simulink model "code_gen_HeadingHold"  (Simulink 7.5)
settings: Solver=FixedStepDiscrete  SolverMode=SingleTasking  StartTime=0.0  StopTime=10.0  FixedStep=0.01  RelTol=1e-3
InitFcn:
  | boat_constants
values from neighbouring files (symbols this model uses):
  figure8_waypoints = int32([ ... (first row only)    [boat_constants.m]
  OC2max = 49999    [boat_constants.m]    (also in simulation_constants.m)
  sampling_waypoints = int32([ ... (first row only)    [boat_constants.m]
  T_step = 0.01    [boat_constants.m]    (also in common.m)
  test_waypoints = int32([ ... (first row only)    [boat_constants.m]
undefined symbols (not defined in the file or in its folder): clearGpsData, clearSensorData, cpInitCommunications, DataEEInitAndClear, DataEEWrite, DiscIntNeverNeededParam, ecan1_buffered_transmit_matlab, ecan1_error_status_matlab, ecan1_init, ecan1_receive_matlab, getGpsData, getSensorData, Init_onlyOnce, Init_Reset, initCalibrationRange, initGps, processNewCommData, processNewGpsData, setHilMode, u1, u2, uart1EnqueueStateData, uart2EnqueueActuatorData, y1
libraries: simulink x85, dsPICdrivers x44, uSimLib x6, simulink_need_slupdate x4, aerolibconvert2 x2
(part 5 of 6)

== system code_gen_HeadingHold/Controller/Autonomous Controller/Throttle Command/Mux Everything/Build speed command ==
  CC : Inport  OutDataType=sfix(16)  OutScaling=2^0
  Constant : Constant  OutDataTypeMode=uint8  OutDataType=sfix(16)  OutScaling=2^0  OutDataTypeStr=uint8
  Constant1 : Constant  Value=0  OutDataTypeMode=uint8  OutDataType=sfix(16)  OutScaling=2^0  OutDataTypeStr=uint8
  Constant2 : Constant  Value=0  OutDataTypeMode=uint8  OutDataType=sfix(16)  OutScaling=2^0  OutDataTypeStr=uint8
  Constant3 : Constant  Value=5  OutDataTypeMode=uint8  OutDataType=sfix(16)  OutScaling=2^0  OutDataTypeStr=uint8
  Mux : Mux  Inputs=5
  uint16 to uchar : Subsystem  AncestorBlock=uSimLib/Conversions/uint16 to uchar
  msg : Outport  OutDataType=sfix(16)  OutScaling=2^0
  wires:
  uint16 to uchar/1(uchar) -> Mux/3
  Constant/1 -> Mux/1
  Constant3/1 -> Mux/2
  Mux/1 -> msg/1
  Constant1/1 -> Mux/4
  Constant2/1 -> Mux/5
  CC/1 -> uint16 to uchar/1(ushort)

== system code_gen_HeadingHold/Controller/RC Inputs/Map PWM values to Actuator Signals/Throttle Command/Mux Everything ==
  speed : Inport  OutDataType=sfix(16)  OutScaling=2^0
  enable : Inport  Port=2  OutDataType=sfix(16)  OutScaling=2^0
  Throttle : Inport  Port=3  OutDataType=sfix(16)  OutScaling=2^0
  0x300 : Constant  Value=768  OutDataTypeMode=uint32  OutDataType=sfix(16)  OutScaling=2^0  OutDataTypeStr=uint32
  0x301 : Constant  Value=769  OutDataTypeMode=uint32  OutDataType=sfix(16)  OutScaling=2^0  OutDataTypeStr=uint32
  Build speed command : Subsystem
  Enable motor : Constant  Value=[0 0 0 0 32 0]  OutDataTypeMode=uint8  OutDataType=sfix(16)  OutScaling=2^0  OutDataTypeStr=uint8
  Message Length1 : Probe  ProbeSampleTime=off  ProbeComplexSignal=off  ProbeWidthDataType=uint8
  Switch : Switch  Criteria=u2 ~= 0  Threshold=1
  Switch1 : Switch  Criteria=u2 ~= 0  OutDataType=fixdt(1, 16)  OutScaling=2^0
  iden : Outport  OutDataType=sfix(16)  OutScaling=2^0
  data : Outport  Port=2  OutDataType=sfix(16)  OutScaling=2^0
  size : Outport  Port=3  OutDataType=sfix(16)  OutScaling=2^0
  trig : Outport  Port=4  OutDataType=sfix(16)  OutScaling=2^0
  wires:
  Throttle/1 -> Build speed command/1(CC)
  Message Length1/1 -> size/1
  0x301/1 -> Switch/3
  Switch1/1 -> Message Length1/1, data/1
  0x300/1 -> Switch/1
  enable/1 -> Switch/2, Switch1/2
  speed/1 -> trig/1
  Enable motor/1 -> Switch1/1
  Build speed command/1(msg) -> Switch1/3
  Switch/1 -> iden/1

== system code_gen_HeadingHold/Controller/RC Inputs/Map PWM values to Actuator Signals/Throttle Command/Trigger Events ==
  Throttle : Inport  OutDataType=sfix(16)  OutScaling=2^0
  Data Type Conversion3 : DataTypeConversion  OutDataTypeMode=boolean  OutDataType=sfix(16)  OutScaling=2^0  OutDataTypeStr=boolean
  Detect Change : simulink/Logic and Bit Operations/Detect Change  SystemSampleTime=-1  vinit=0
  Shift Arithmetic : simulink/Logic and Bit Operations/Shift Arithmetic  SystemSampleTime=-1  nBitShiftRight=2  nBinPtShiftRight=0
  Weighted Moving Average : simulink_need_slupdate/Weighted Moving Average  mgainval=[.5 .5]  vinit=0.0  samptime=-1  OutDataTypeStr=Inherit: Inherit via back propagation  OutDataType=sfix(16)  OutScaling=2^-10  DoSatur=off  GainDataType=uint(16)  MatRadixGroup=Best Precision: Matrix-wise  GainScaling=2^-10
  Change Speed : Outport  OutDataType=sfix(16)  OutScaling=2^0
  wires:
  Throttle/1 -> Shift Arithmetic/1
  Detect Change/1 -> Data Type Conversion3/1
  Data Type Conversion3/1 -> Change Speed/1
  Weighted Moving Average/1 -> Detect Change/1
  Shift Arithmetic/1 -> Weighted Moving Average/1

== system code_gen_HeadingHold/Controller/Radio Control Inputs1/Calibration/Update range from input/If Action Subsystem ==
  In1 : Inport  OutDataType=fixdt(1, 16)  OutScaling=2^0
  Action Port : ActionPort  ActionType=then
  Out1 : Outport  OutDataType=fixdt(1, 16)  OutScaling=2^0
  wires:
  In1/1 -> Out1/1

== system code_gen_HeadingHold/Controller/Radio Control Inputs1/Calibration/Update range from input/If Action Subsystem1 ==
  In1 : Inport  OutDataType=fixdt(1, 16)  OutScaling=2^0
  Action Port : ActionPort  ActionType=else
  Out1 : Outport  OutDataType=fixdt(1, 16)  OutScaling=2^0
  wires:
  In1/1 -> Out1/1

== system code_gen_HeadingHold/Controller/Radio Control Inputs1/Calibration/Update range from input/If Action Subsystem2 ==
  In1 : Inport  OutDataType=fixdt(1, 16)  OutScaling=2^0
  Action Port : ActionPort  ActionType=then
  Out1 : Outport  OutDataType=fixdt(1, 16)  OutScaling=2^0
  wires:
  In1/1 -> Out1/1

== system code_gen_HeadingHold/Controller/Radio Control Inputs1/Calibration/Update range from input/If Action Subsystem3 ==
  In1 : Inport  OutDataType=fixdt(1, 16)  OutScaling=2^0
  Action Port : ActionPort  ActionType=else
  Out1 : Outport  OutDataType=fixdt(1, 16)  OutScaling=2^0
  wires:
  In1/1 -> Out1/1

== system code_gen_HeadingHold/Controller/Radio Control Inputs1/Calibration/Update range from input1/If Action Subsystem ==
  In1 : Inport  OutDataType=fixdt(1, 16)  OutScaling=2^0
  Action Port : ActionPort  ActionType=then
  Out1 : Outport  OutDataType=fixdt(1, 16)  OutScaling=2^0
  wires:
  In1/1 -> Out1/1

== system code_gen_HeadingHold/Controller/Radio Control Inputs1/Calibration/Update range from input1/If Action Subsystem1 ==
  In1 : Inport  OutDataType=fixdt(1, 16)  OutScaling=2^0
  Action Port : ActionPort  ActionType=else
  Out1 : Outport  OutDataType=fixdt(1, 16)  OutScaling=2^0
  wires:
  In1/1 -> Out1/1

== system code_gen_HeadingHold/Controller/Radio Control Inputs1/Calibration/Update range from input1/If Action Subsystem2 ==
  In1 : Inport  OutDataType=fixdt(1, 16)  OutScaling=2^0
  Action Port : ActionPort  ActionType=then
  Out1 : Outport  OutDataType=fixdt(1, 16)  OutScaling=2^0
  wires:
  In1/1 -> Out1/1

== system code_gen_HeadingHold/Controller/Radio Control Inputs1/Calibration/Update range from input1/If Action Subsystem3 ==
  In1 : Inport  OutDataType=fixdt(1, 16)  OutScaling=2^0
  Action Port : ActionPort  ActionType=else
  Out1 : Outport  OutDataType=fixdt(1, 16)  OutScaling=2^0
  wires:
  In1/1 -> Out1/1

== system code_gen_HeadingHold/Controller/Radio Control Inputs1/Calibration/Update range from input2/If Action Subsystem ==
  In1 : Inport  OutDataType=fixdt(1, 16)  OutScaling=2^0
  Action Port : ActionPort  ActionType=then
  Out1 : Outport  OutDataType=fixdt(1, 16)  OutScaling=2^0
  wires:
  In1/1 -> Out1/1

== system code_gen_HeadingHold/Controller/Radio Control Inputs1/Calibration/Update range from input2/If Action Subsystem1 ==
  In1 : Inport  OutDataType=fixdt(1, 16)  OutScaling=2^0
  Action Port : ActionPort  ActionType=else
  Out1 : Outport  OutDataType=fixdt(1, 16)  OutScaling=2^0
  wires:
  In1/1 -> Out1/1

== system code_gen_HeadingHold/Controller/Radio Control Inputs1/Calibration/Update range from input2/If Action Subsystem2 ==
  In1 : Inport  OutDataType=fixdt(1, 16)  OutScaling=2^0
  Action Port : ActionPort  ActionType=then
  Out1 : Outport  OutDataType=fixdt(1, 16)  OutScaling=2^0
  wires:
  In1/1 -> Out1/1

== system code_gen_HeadingHold/Controller/Radio Control Inputs1/Calibration/Update range from input2/If Action Subsystem3 ==
  In1 : Inport  OutDataType=fixdt(1, 16)  OutScaling=2^0
  Action Port : ActionPort  ActionType=else
  Out1 : Outport  OutDataType=fixdt(1, 16)  OutScaling=2^0
  wires:
  In1/1 -> Out1/1

== system code_gen_HeadingHold/Controller/Radio Control Inputs1/Detect calibration trigger/State outputs/If Action Subsystem1 ==
  Action Port : ActionPort  ActionType=then
  Constant1 : Constant  Value=false  OutDataType=fixdt(1, 16)  OutScaling=2^0  OutDataTypeStr=Inherit: Inherit via back propagation
  LED : Outport  OutDataType=fixdt(1, 16)  OutScaling=2^0  InitialOutput=false
  wires:
  Constant1/1 -> LED/1

== system code_gen_HeadingHold/Controller/Radio Control Inputs1/Detect calibration trigger/State outputs/If Action Subsystem2 ==
  Action Port : ActionPort  ActionType=else
  Constant1 : Constant  Value=false  OutDataType=fixdt(1, 16)  OutScaling=2^0  OutDataTypeStr=Inherit: Inherit via back propagation
  LED : Outport  OutDataType=fixdt(1, 16)  OutScaling=2^0  InitialOutput=false
  wires:
  Constant1/1 -> LED/1

== system code_gen_HeadingHold/Controller/Radio Control Inputs1/Detect calibration trigger/State outputs/If Action Subsystem3 ==
  Pulse : Inport
  Action Port : ActionPort  ActionType=elseif
  LED : Outport  OutDataType=fixdt(1, 16)  OutScaling=2^0  InitialOutput=false
  wires:
  Pulse/1 -> LED/1

== system code_gen_HeadingHold/Controller/Radio Control Inputs1/Detect calibration trigger/State outputs/If Action Subsystem4 ==
  Action Port : ActionPort  ActionType=elseif
  Constant1 : Constant  Value=true  OutDataType=fixdt(1, 16)  OutScaling=2^0  OutDataTypeStr=Inherit: Inherit via back propagation
  LED : Outport  OutDataType=fixdt(1, 16)  OutScaling=2^0  InitialOutput=false
  wires:
  Constant1/1 -> LED/1

== system code_gen_HeadingHold/Controller/Radio Control Inputs1/If Action Subsystem1/Add 8% center deadband/If Action Subsystem ==
  In1 : Inport  OutDataType=fixdt(1, 16)  OutScaling=2^0
  Action Port : ActionPort  ActionType=else
  Out1 : Outport  OutDataType=fixdt(1, 16)  OutScaling=2^0
  wires:
  In1/1 -> Out1/1

== system code_gen_HeadingHold/Controller/Radio Control Inputs1/If Action Subsystem1/Add 8% center deadband/If Action Subsystem1 ==
  Action Port : ActionPort  ActionType=then
  Constant : Constant  Value=0  OutDataType=fixdt(1, 16)  OutScaling=2^0  OutDataTypeStr=Inherit: Inherit via back propagation
  Out1 : Outport  OutDataType=fixdt(1, 16)  OutScaling=2^0  InitialOutput=50
  wires:
  Constant/1 -> Out1/1

== system code_gen_HeadingHold/Controller/Radio Control Inputs1/If Action Subsystem3/Add 5% deadband about 0/If Action Subsystem ==
  In1 : Inport  OutDataType=fixdt(1, 16)  OutScaling=2^0
  Action Port : ActionPort  ActionType=else
  Out1 : Outport  OutDataType=fixdt(1, 16)  OutScaling=2^0
  wires:
  In1/1 -> Out1/1

== system code_gen_HeadingHold/Controller/Radio Control Inputs1/If Action Subsystem3/Add 5% deadband about 0/If Action Subsystem1 ==
  Action Port : ActionPort  ActionType=then
  Constant : Constant  Value=0  OutDataType=fixdt(1, 16)  OutScaling=2^0  OutDataTypeStr=Inherit: Inherit via back propagation
  Out1 : Outport  OutDataType=fixdt(1, 16)  OutScaling=2^0  InitialOutput=0
  wires:
  Constant/1 -> Out1/1

== system code_gen_HeadingHold/Controller/Radio Control Inputs1/If Action Subsystem5/Add 8% center deadband/If Action Subsystem ==
  In1 : Inport  OutDataType=fixdt(1, 16)  OutScaling=2^0
  Action Port : ActionPort  ActionType=else
  Out1 : Outport  OutDataType=fixdt(1, 16)  OutScaling=2^0
  wires:
  In1/1 -> Out1/1

== system code_gen_HeadingHold/Controller/Radio Control Inputs1/If Action Subsystem5/Add 8% center deadband/If Action Subsystem1 ==
  Action Port : ActionPort  ActionType=then
  Constant : Constant  Value=500  OutDataType=fixdt(1, 16)  OutScaling=2^0  OutDataTypeStr=Inherit: Inherit via back propagation
  Out1 : Outport  OutDataType=fixdt(1, 16)  OutScaling=2^0  InitialOutput=50
  wires:
  Constant/1 -> Out1/1

== system code_gen_HeadingHold/Controller/Split trackCommand to singular commands/Countdown timer for trigger/State transitions/Null transition (necessary for merge block) ==
  Action Port : ActionPort  ActionType=else
  Constant1 : Constant  Value=false  OutDataTypeMode=boolean  OutDataType=fixdt(1, 16)  OutScaling=2^0  OutDataTypeStr=boolean
  Constant3 : Constant  Value=false  OutDataTypeMode=boolean  OutDataType=fixdt(1, 16)  OutScaling=2^0  OutDataTypeStr=boolean
  startTimer : Outport  OutDataType=fixdt(1, 16)  OutScaling=2^0  InitialOutput=false
  trigger : Outport  Port=2  OutDataType=fixdt(1, 16)  OutScaling=2^0  InitialOutput=false
  wires:
  Constant3/1 -> startTimer/1
  Constant1/1 -> trigger/1

== system code_gen_HeadingHold/Controller/Split trackCommand to singular commands/Countdown timer for trigger/State transitions/Transition from 0 to 1 ==
  Action Port : ActionPort  ActionType=then
  Constant : Constant  OutDataType=fixdt(1, 16)  OutScaling=2^0  OutDataTypeStr=Inherit: Inherit via back propagation
  Constant2 : Constant  Value=true  OutDataTypeMode=boolean  OutDataType=fixdt(1, 16)  OutScaling=2^0  OutDataTypeStr=boolean
  Constant3 : Constant  Value=false  OutDataTypeMode=boolean  OutDataType=fixdt(1, 16)  OutScaling=2^0  OutDataTypeStr=boolean
  Data Store Write : DataStoreWrite  DataStoreName=timerState  SampleTime=-1
  startTimer : Outport  OutDataType=fixdt(1, 16)  OutScaling=2^0  InitialOutput=true
  trigger : Outport  Port=2  OutDataType=fixdt(1, 16)  OutScaling=2^0  InitialOutput=true
  wires:
  Constant/1 -> Data Store Write/1
  Constant2/1 -> startTimer/1
  Constant3/1 -> trigger/1

== system code_gen_HeadingHold/Controller/Split trackCommand to singular commands/Countdown timer for trigger/State transitions/Transition from 1 to 0 ==
  Action Port : ActionPort  ActionType=elseif
  Constant : Constant  Value=0  OutDataType=fixdt(1, 16)  OutScaling=2^0  OutDataTypeStr=Inherit: Inherit via back propagation
  Constant1 : Constant  Value=false  OutDataTypeMode=boolean  OutDataType=fixdt(1, 16)  OutScaling=2^0  OutDataTypeStr=boolean
  Constant3 : Constant  Value=false  OutDataTypeMode=boolean  OutDataType=fixdt(1, 16)  OutScaling=2^0  OutDataTypeStr=boolean
  Data Store Write : DataStoreWrite  DataStoreName=timerState  SampleTime=-1
  startTimer : Outport  OutDataType=fixdt(1, 16)  OutScaling=2^0  InitialOutput=false
  trigger : Outport  Port=2  OutDataType=fixdt(1, 16)  OutScaling=2^0  InitialOutput=false
  wires:
  Constant/1 -> Data Store Write/1
  Constant3/1 -> startTimer/1
  Constant1/1 -> trigger/1

== system code_gen_HeadingHold/Controller/Split trackCommand to singular commands/Countdown timer for trigger/State transitions/Transition from 1 to 2 ==
  Action Port : ActionPort  ActionType=elseif
  Constant : Constant  Value=2  OutDataType=fixdt(1, 16)  OutScaling=2^0  OutDataTypeStr=Inherit: Inherit via back propagation
  Constant1 : Constant  Value=true  OutDataTypeMode=boolean  OutDataType=fixdt(1, 16)  OutScaling=2^0  OutDataTypeStr=boolean
  Constant3 : Constant  Value=false  OutDataTypeMode=boolean  OutDataType=fixdt(1, 16)  OutScaling=2^0  OutDataTypeStr=boolean
  Data Store Write : DataStoreWrite  DataStoreName=timerState  SampleTime=-1
  startTimer : Outport  OutDataType=fixdt(1, 16)  OutScaling=2^0  InitialOutput=false
  trigger : Outport  Port=2  OutDataType=fixdt(1, 16)  OutScaling=2^0  InitialOutput=false
  wires:
  Constant/1 -> Data Store Write/1
  Constant3/1 -> startTimer/1
  Constant1/1 -> trigger/1

== system code_gen_HeadingHold/Controller/Split trackCommand to singular commands/Countdown timer for trigger/State transitions/Transition from 2 to 0 ==
  Action Port : ActionPort  ActionType=elseif
  Constant : Constant  Value=0  OutDataType=fixdt(1, 16)  OutScaling=2^0  OutDataTypeStr=Inherit: Inherit via back propagation
  Constant1 : Constant  Value=false  OutDataTypeMode=boolean  OutDataType=fixdt(1, 16)  OutScaling=2^0  OutDataTypeStr=boolean
  Constant3 : Constant  Value=false  OutDataTypeMode=boolean  OutDataType=fixdt(1, 16)  OutScaling=2^0  OutDataTypeStr=boolean
  Data Store Write : DataStoreWrite  DataStoreName=timerState  SampleTime=-1
  startTimer : Outport  OutDataType=fixdt(1, 16)  OutScaling=2^0  InitialOutput=false
  trigger : Outport  Port=2  OutDataType=fixdt(1, 16)  OutScaling=2^0  InitialOutput=false
  wires:
  Constant/1 -> Data Store Write/1
  Constant3/1 -> startTimer/1
  Constant1/1 -> trigger/1

== system code_gen_HeadingHold/Controller/Split trackCommand to singular commands/Countdown timer for trigger1/State transitions/Null transition (necessary for merge block) ==
  Action Port : ActionPort  ActionType=else
  Constant1 : Constant  Value=false  OutDataTypeMode=boolean  OutDataType=fixdt(1, 16)  OutScaling=2^0  OutDataTypeStr=boolean
  Constant3 : Constant  Value=false  OutDataTypeMode=boolean  OutDataType=fixdt(1, 16)  OutScaling=2^0  OutDataTypeStr=boolean
  startTimer : Outport  OutDataType=fixdt(1, 16)  OutScaling=2^0  InitialOutput=false
  trigger : Outport  Port=2  OutDataType=fixdt(1, 16)  OutScaling=2^0  InitialOutput=false
  wires:
  Constant1/1 -> trigger/1
  Constant3/1 -> startTimer/1

== system code_gen_HeadingHold/Controller/Split trackCommand to singular commands/Countdown timer for trigger1/State transitions/Transition from 0 to 1 ==
  Action Port : ActionPort  ActionType=then
  Constant : Constant  OutDataType=fixdt(1, 16)  OutScaling=2^0  OutDataTypeStr=Inherit: Inherit via back propagation
  Constant2 : Constant  Value=true  OutDataTypeMode=boolean  OutDataType=fixdt(1, 16)  OutScaling=2^0  OutDataTypeStr=boolean
  Constant3 : Constant  Value=false  OutDataTypeMode=boolean  OutDataType=fixdt(1, 16)  OutScaling=2^0  OutDataTypeStr=boolean
  Data Store Write : DataStoreWrite  DataStoreName=timerState2  SampleTime=-1
  startTimer : Outport  OutDataType=fixdt(1, 16)  OutScaling=2^0  InitialOutput=true
  trigger : Outport  Port=2  OutDataType=fixdt(1, 16)  OutScaling=2^0  InitialOutput=true
  wires:
  Constant3/1 -> trigger/1
  Constant2/1 -> startTimer/1
  Constant/1 -> Data Store Write/1

== system code_gen_HeadingHold/Controller/Split trackCommand to singular commands/Countdown timer for trigger1/State transitions/Transition from 1 to 0 ==
  Action Port : ActionPort  ActionType=elseif
  Constant : Constant  Value=0  OutDataType=fixdt(1, 16)  OutScaling=2^0  OutDataTypeStr=Inherit: Inherit via back propagation
  Constant1 : Constant  Value=false  OutDataTypeMode=boolean  OutDataType=fixdt(1, 16)  OutScaling=2^0  OutDataTypeStr=boolean
  Constant3 : Constant  Value=false  OutDataTypeMode=boolean  OutDataType=fixdt(1, 16)  OutScaling=2^0  OutDataTypeStr=boolean
  Data Store Write : DataStoreWrite  DataStoreName=timerState2  SampleTime=-1
  startTimer : Outport  OutDataType=fixdt(1, 16)  OutScaling=2^0  InitialOutput=false
  trigger : Outport  Port=2  OutDataType=fixdt(1, 16)  OutScaling=2^0  InitialOutput=false
  wires:
  Constant1/1 -> trigger/1
  Constant3/1 -> startTimer/1
  Constant/1 -> Data Store Write/1

== system code_gen_HeadingHold/Controller/Split trackCommand to singular commands/Countdown timer for trigger1/State transitions/Transition from 1 to 2 ==
  Action Port : ActionPort  ActionType=elseif
  Constant : Constant  Value=2  OutDataType=fixdt(1, 16)  OutScaling=2^0  OutDataTypeStr=Inherit: Inherit via back propagation
  Constant1 : Constant  Value=true  OutDataTypeMode=boolean  OutDataType=fixdt(1, 16)  OutScaling=2^0  OutDataTypeStr=boolean
  Constant3 : Constant  Value=false  OutDataTypeMode=boolean  OutDataType=fixdt(1, 16)  OutScaling=2^0  OutDataTypeStr=boolean
  Data Store Write : DataStoreWrite  DataStoreName=timerState2  SampleTime=-1
  startTimer : Outport  OutDataType=fixdt(1, 16)  OutScaling=2^0  InitialOutput=false
  trigger : Outport  Port=2  OutDataType=fixdt(1, 16)  OutScaling=2^0  InitialOutput=false
  wires:
  Constant1/1 -> trigger/1
  Constant3/1 -> startTimer/1
  Constant/1 -> Data Store Write/1

== system code_gen_HeadingHold/Controller/Split trackCommand to singular commands/Countdown timer for trigger1/State transitions/Transition from 2 to 0 ==
  Action Port : ActionPort  ActionType=elseif
  Constant : Constant  Value=0  OutDataType=fixdt(1, 16)  OutScaling=2^0  OutDataTypeStr=Inherit: Inherit via back propagation
  Constant1 : Constant  Value=false  OutDataTypeMode=boolean  OutDataType=fixdt(1, 16)  OutScaling=2^0  OutDataTypeStr=boolean
  Constant3 : Constant  Value=false  OutDataTypeMode=boolean  OutDataType=fixdt(1, 16)  OutScaling=2^0  OutDataTypeStr=boolean
  Data Store Write : DataStoreWrite  DataStoreName=timerState2  SampleTime=-1
  startTimer : Outport  OutDataType=fixdt(1, 16)  OutScaling=2^0  InitialOutput=false
  trigger : Outport  Port=2  OutDataType=fixdt(1, 16)  OutScaling=2^0  InitialOutput=false
  wires:
  Constant1/1 -> trigger/1
  Constant3/1 -> startTimer/1
  Constant/1 -> Data Store Write/1

== system code_gen_HeadingHold/Controller/Autonomous Controller/State Keeper & Estimator/GPS Estimator/Subsystem/Reorder ==
  In1 : Inport
  Angle Conversion : uSimLib/Conversions/Angle Conversion  SystemSampleTime=-1  iu=deg  ou=rad
  Angle Conversion1 : uSimLib/Conversions/Angle Conversion  SystemSampleTime=-1  iu=deg  ou=rad
  Bias : Bias  Bias=2000
  Bus Selector : BusSelector  OutputSignals=latitude,longitude,year,month,day,hour,minute,second
  Constant : Constant  Value=0  OutDataTypeMode=single  OutDataType=fixdt(1, 16)  OutScaling=2^0  OutDataTypeStr=single
  Data Type Conversion{1..8} (8 alike) : DataTypeConversion  OutDataTypeMode=single  OutDataType=fixdt(1, 16)  OutScaling=2^0  OutDataTypeStr=single
  Mux : Mux  Inputs=7
  Mux1 : Mux  Inputs=3
  Phase shift2 : Constant  Value=-8  OutDataTypeMode=single  OutDataType=sfix(16)  OutScaling=2^0  OutDataTypeStr=single
  Scope : Scope
  pos : Outport
  time : Outport  Port=2
  wires:
  Bus Selector/1 -> Data Type Conversion8/1  "<latitude>"
  Bus Selector/2 -> Data Type Conversion7/1  "<longitude>"
  Data Type Conversion1/1 -> Bias/1
  Bias/1 -> Mux/1
  Data Type Conversion2/1 -> Mux/2
  Bus Selector/3 -> Data Type Conversion1/1  "<year>"
  Bus Selector/4 -> Data Type Conversion2/1  "<month>"
  Bus Selector/5 -> Data Type Conversion3/1  "<day>"
  Bus Selector/6 -> Data Type Conversion4/1  "<hour>"
  Bus Selector/7 -> Data Type Conversion5/1  "<minute>"
  Bus Selector/8 -> Data Type Conversion6/1  "<second>"
  Data Type Conversion3/1 -> Mux/3
  Data Type Conversion4/1 -> Mux/4
  Data Type Conversion5/1 -> Mux/5
  Data Type Conversion6/1 -> Mux/6
  Phase shift2/1 -> Mux/7
  In1/1 -> Bus Selector/1
  Mux/1 -> time/1
  Angle Conversion/1 -> Scope/1, Mux1/1
  Angle Conversion1/1 -> Mux1/2
  Constant/1 -> Mux1/3
  Mux1/1 -> pos/1
  Data Type Conversion7/1 -> Angle Conversion1/1
  Data Type Conversion8/1 -> Angle Conversion/1

== system code_gen_HeadingHold/Controller/Autonomous Controller/Throttle Command/Mux Everything/Build speed command/uint16 to uchar ==
  ushort : Inport
  Data Type Conversion : DataTypeConversion  OutDataTypeMode=uint16  OutDataType=fixdt(1, 16)  OutScaling=2^0  OutDataTypeStr=uint16  ConvertRealWorld=Stored Integer (SI)  RndMeth=Simplest
  Extract Bits1 : simulink/Logic and Bit Operations/Extract Bits  SystemSampleTime=-1  bitsToExtract=Upper half  numBits=8  bitIdxRange=[0 7]  outScalingMode=Treat bit field as an integer
  Extract Bits2 : simulink/Logic and Bit Operations/Extract Bits  SystemSampleTime=-1  bitsToExtract=Lower half  numBits=8  bitIdxRange=[0 7]  outScalingMode=Treat bit field as an integer
  Mux : Mux  Inputs=2
  uchar : Outport  OutDataType=fixdt(1, 16)  OutScaling=2^0
  wires:
  Mux/1 -> uchar/1
  Extract Bits2/1 -> Mux/2
  Extract Bits1/1 -> Mux/1
  ushort/1 -> Data Type Conversion/1
  Data Type Conversion/1 -> Extract Bits1/1, Extract Bits2/1

== system code_gen_HeadingHold/Controller/RC Inputs/Map PWM values to Actuator Signals/Throttle Command/Mux Everything/Build speed command ==
  CC : Inport  OutDataType=sfix(16)  OutScaling=2^0
  Constant : Constant  OutDataTypeMode=uint8  OutDataType=sfix(16)  OutScaling=2^0  OutDataTypeStr=uint8
  Constant1 : Constant  Value=0  OutDataTypeMode=uint8  OutDataType=sfix(16)  OutScaling=2^0  OutDataTypeStr=uint8
  Constant2 : Constant  Value=0  OutDataTypeMode=uint8  OutDataType=sfix(16)  OutScaling=2^0  OutDataTypeStr=uint8
  Constant3 : Constant  Value=5  OutDataTypeMode=uint8  OutDataType=sfix(16)  OutScaling=2^0  OutDataTypeStr=uint8
  Data Type Conversion1 : DataTypeConversion  OutDataTypeMode=uint8  OutDataType=sfix(16)  OutScaling=2^0  OutDataTypeStr=uint8  ConvertRealWorld=Stored Integer (SI)
  Data Type Conversion2 : DataTypeConversion  OutDataTypeMode=uint8  OutDataType=sfix(16)  OutScaling=2^0  OutDataTypeStr=uint8  ConvertRealWorld=Stored Integer (SI)
  Data Type Conversion3 : DataTypeConversion  OutDataTypeMode=uint16  OutDataType=sfix(16)  OutScaling=2^0  OutDataTypeStr=uint16  ConvertRealWorld=Stored Integer (SI)
  Extract Bits : simulink/Logic and Bit Operations/Extract Bits  SystemSampleTime=-1  bitsToExtract=Upper half  numBits=8  bitIdxRange=[24 31]  outScalingMode=Treat bit field as an integer
  Extract Bits1 : simulink/Logic and Bit Operations/Extract Bits  SystemSampleTime=-1  bitsToExtract=Lower half  numBits=8  bitIdxRange=[16 23]  outScalingMode=Treat bit field as an integer
  myMux : Stateflow chart  TreatAsAtomicUnit=on
  msg : Outport  OutDataType=sfix(16)  OutScaling=2^0
  wires:
  Constant2/1 -> myMux/6(u6)
  myMux/1(y) -> msg/1
  Constant3/1 -> myMux/2(u2)
  Constant/1 -> myMux/1(u1)
  Constant1/1 -> myMux/5(u5)
  Extract Bits1/1 -> Data Type Conversion2/1
  Extract Bits/1 -> Data Type Conversion1/1
  CC/1 -> Data Type Conversion3/1
  Data Type Conversion1/1 -> myMux/3(u3)
  Data Type Conversion2/1 -> myMux/4(u4)
  Data Type Conversion3/1 -> Extract Bits1/1, Extract Bits/1

== matlab function Controller/Autonomous Controller/State Keeper & Estimator/GPS Estimator/Calculate local position via velocity integral between true GPS updates ==
  data: latLonAlt input single size=[3 1]; localPosition output single; newData input boolean size=1; reset input boolean size=1; resetIntegrator output boolean size=1
function [localPosition,resetIntegrator] = estimateGPS(latLonAlt, newData, reset)
%#eml
% INPUTS:
% latLonAlt - the latitude, longitude, and altitude of the vehicle from GPS
% newData - A boolean signal specifying whether latLonAlt holds new data
% reset - A global reset boolean trigger.

% OUTPUTS:
% localPosition is the local position of the vehicle in relation to a recorded
% starting location in North-East-Down coordinates.
% resetIntegrator will reset the velocity integrator that's calculating the
% local position in between GPS reads.

persistent startingPosition lastKnownPosition newDataCounter;

% Reset everything on first startup or when a global reset is triggered
if isempty(startingPosition) || reset
    startingPosition = zeros(3, 1, 'single');
end
if isempty(lastKnownPosition) || reset
    lastKnownPosition = zeros(3, 1, 'single');
end
if isempty(newDataCounter) || reset
    newDataCounter = zeros(1, 1, 'uint8');
end

% Reset the integrator if a global reset is called
if reset
    resetIntegrator = true;
else
    resetIntegrator = false;
end

% Wait for 5 valid GPS inputs before latching a starting point
if newDataCounter < 5
    % Check that we have valid data before latching it.
    if newData && latLonAlt(1) ~= 0 && latLonAlt(2) ~= 0
        newDataCounter = newDataCounter + 1;
        startingPosition = latLonAlt;
    end
    
    % We output all 0s while we're waiting
    localPosition = zeros(3, 1, 'single');
else
    % Latch a new position if one's been received. Also reset the integrator
    % for this timestep as we have a "truth" position now.
    if newData
        lastKnownPosition = latLonAlt;
        resetIntegrator = true;
    end
    
    % Calculate the difference between the starting position and the last
    % known position.
    localPosition = dg2lg(startingPosition, latLonAlt);
end

% Not certain how this works or where I got it from.
function out = dg2lg(u1, u2)

dlat = (u2(1) - u1(1))*pi/180;
dlon = (u2(2) - u1(2))*pi/180;
lat = u1(1)*pi/180;
h = u2(3);
a = 6378137;
e2 = 0.00669437999014;

v=a./sqrt(1-e2.*sin(lat).^2);
r=v.*(1-e2)./(1-e2.*sin(lat).^2);
dx=dlat.*(r+h);
dy=dlon.*cos(lat).*(v+h);

% Map into North-East-Down coordinates
out = [dx; dy; 0];

== matlab function Transmit actuator data/Package and Transmit Sensor Struct/Pack ==
  data: r_en input double; y output double; r_dir input double; r_up input double; r_per input double; b_en input double; b_dir input double; t_id input double; t_data input double; t_size input double; t_trig input double; time input double; rudderAngle input double; sensorOverride input double
function y = fcn(r_en, r_dir, r_up, r_per, b_en, b_dir, t_id, t_data, t_size, t_trig, time, rudderAngle, sensorOverride)
%#eml

y = zeros(27, 1, 'uint8');
y(1) = uint8(r_en);
y(2) = uint8(r_dir);
y(3) = uint8(bitand(r_up,hex2dec('FF')));
y(4) = uint8(bitand(bitshift(r_up,-8),hex2dec('FF')));
y(5) = uint8(bitand(r_per,hex2dec('FF')));
y(6) = uint8(bitand(bitshift(r_per,-8),hex2dec('FF')));
y(7) = uint8(b_en);
y(8) = uint8(b_dir);
y(9) = uint8(bitand(t_id,hex2dec('FF')));
y(10) = uint8(bitand(bitshift(t_id,-8),hex2dec('FF')));
y(11) = uint8(bitand(bitshift(t_id,-16),hex2dec('FF')));
y(12) = uint8(bitand(bitshift(t_id,-24),hex2dec('FF')));
y(13:18) = t_data(1:6);
y(19) = t_size;
y(20) = uint8(t_trig);
y(21) = uint8(bitand(typecast(time,'uint16'),hex2dec('FF')));
y(22) = uint8(bitand(bitshift(typecast(time,'uint16'),-8),hex2dec('FF')));
y(23) = uint8(bitand(typecast(rudderAngle,'uint32'),hex2dec('FF')));
y(24) = uint8(bitand(bitshift(typecast(rudderAngle,'uint32'),-8),hex2dec('FF')));
y(25) = uint8(bitand(bitshift(typecast(rudderAngle,'uint32'),-16),hex2dec('FF')));
y(26) = uint8(bitand(bitshift(typecast(rudderAngle,'uint32'),-24),hex2dec('FF')));
y(27) = sensorOverride

== matlab function Transmit actuator data/Package and Transmit Sensor Struct/Build HIL sentence/Pack ==
  data: a input double; y output double; b input double; c input double; d input double; e input double; f input double
function y = fcn(a, b, c, d, e, f)
%#eml

y = zeros(34, 1, 'uint8');
y(1) = a;
y(2) = b;
y(3:31) = c;
y(32) = d;
y(33) = e;
y(34) = f;

== matlab function Controller/RC Inputs/Map PWM values to Actuator Signals/Throttle Command/Mux Everything/Build speed command/myMux ==
  data: u1 input double; y output double; u2 input double; u3 input double; u4 input double; u5 input double; u6 input double
function y = myMux(u1, u2, u3, u4, u5, u6)
y = [u1(1); u2(1); u3(1); u4(1); u5(1); u6(1);];

== matlab function Sensor Inputs/Parse for HIL data/Unpack sensor data ==
  data: u input uint8; throttle output double; latitude output double; longitude output double; altitude output double; year output double; month output double; day output double; hour output double; minute output double; second output double; cog output double; sog output double; newGpsData output double; rudderPosition output double; rudderStarboardLimit output double; rudderPortLimit output double; ballastPosition output double; ballastStarboardLimit output double; ballastPortLimit output double; timestamp output double; newData output double
function [throttle, latitude, longitude, altitude, year, month, day, hour, minute, second, cog, sog, newGpsData, rudderPosition, rudderStarboardLimit, rudderPortLimit, ballastPosition, ballastStarboardLimit, ballastPortLimit, timestamp, newData] = unpack(u)
%#eml

throttle = typecast(u(1:2), 'int16');
latitude = typecast(u(3:6), 'single');
longitude = typecast(u(7:10), 'single');
altitude = typecast(u(11:14), 'single');
year = u(15);
month = u(16);
day = u(17);
hour = u(18);
minute = u(19);
second = u(20);
cog = typecast(u(21:24), 'single');
sog = typecast(u(25:28), 'single');
newGpsData = u(29);
rudderPosition = typecast(u(30:31), 'uint16');
rudderStarboardLimit = u(32);
rudderPortLimit = u(33);
ballastPosition = typecast(u(34:35), 'uint16');
ballastStarboardLimit = u(36);
ballastPortLimit = u(37);
timestamp = typecast(u(38:39), 'int16');
newData = u(40);

== matlab function Controller/Autonomous Controller/Rudder Command/Latch first signal ==
  data: haveHeading output double; heading input single size=1; latchedHeading output single size=1; reset input boolean size=1
function [haveHeading,latchedHeading] = latchFirstHeading(heading, reset)
%#eml

% This Matlab function latches its input and only resets it when a reset is triggered.

persistent storedHeading haveData;

% Reset everything on first startup or when a global reset is triggered
if isempty(storedHeading) || reset
    storedHeading = single(0);
    haveData = false;
end

if ~haveData && ~reset
    storedHeading = heading;
    haveData = true;
end

haveHeading = haveData;
latchedHeading = storedHeading;

== matlab function Actuator Outputs/To Drive Motor/myMux ==
  data: u1 input double; y output double; u2 input double; u3 input double; u4 input double; u5 input double
function y = myMux(u1, u2, u3, u4, u5)
u5_u16 = uint16(u5);
y = uint16([u1(1); u2(1); u3(1); u4(1); 0; 0; 0; 0;]);

len = length(u5);
if len > 1
    y(5) = bitor(bitshift(u5_u16(1),8),u5_u16(2));
elseif len > 0
    y(5) = u5_u16(1);
end
if len > 3
    y(6) = bitor(bitshift(u5_u16(3),8),u5_u16(4));
elseif len > 2
    y(6) = u5_u16(3);
end
if len > 5
    y(7) = bitor(bitshift(u5_u16(5),8),u5_u16(6));
elseif len > 4
    y(7) = u5_u16(5);
end
if len > 7
    y(8) = bitor(bitshift(u5_u16(7),8),u5_u16(8));
elseif len > 6
    y(8) = u5_u16(7);
end

== matlab function Sensor Inputs/GPS/Unpack sensor data ==
  data: latitude output double; longitude output double; altitude output double; year output double; month output double; day output double; hour output double; minute output double; second output double; cog output double; sog output double; u input uint8; hdop output double; fix output double; satellites output double; newGpsData output double
function [latitude, longitude, altitude, year, month, day, hour, minute, second, cog, sog, hdop, fix, satellites, newGpsData] = unpack(u)
%#eml

latitude = typecast(u(1:4), 'single');
longitude = typecast(u(5:8), 'single');
altitude = typecast(u(9:12), 'single');
year = u(13);
month = u(14);
day = u(15);
hour = u(16);
minute = u(17);
second = u(18);
cog = typecast(u(19:22), 'single');
sog = typecast(u(23:26), 'single');
hdop = typecast(u(27:30), 'single');
fix = u(31);
satellites = u(32);
newGpsData = u(33);

== matlab function Controller/Rudder sensor calibration/Convert rudder sensor readings into rudder angle ==
  data: in input uint16; rads output single; port_limit input boolean; starboard_limit input boolean; calibrated output double; reset input double; low_limit output double; high_limit output double
function [rads, calibrated, low_limit, high_limit] = pot_to_rads(in, port_limit, starboard_limit, reset)
%#eml
% This function converts the potentiometer reading from the boat's rudder sensors
% to a value in degrees. It relies on each limit being hit to set the bounds on
% the rudder sensor value and then maps that value from that range into the new
% range of -.07854 to .07854 (+-45 deg). It is loosely based off of the integer
% mapping function at: http://www.arduino.cc/cgi-bin/yabb2/YaBB.pl?num=1289758376

persistent low_side high_side lastInput offset cal
if isempty(low_side) || isempty(high_side) || reset
    low_side = int32(-1);
    high_side = int32(-1);
    lastInput = int32(-10000);
    offset = int32(0);
    cal = false;
end

% Here we track transitions. On a high->low transition start adding 1023
% and on a low->high transition don't add anything. It "centers" the input
% range around 1023.
input = int32(in);
if lastInput == uint32(-10000)
    lastInput = input;
end
jump = input - lastInput;
if jump > 1000
    offset = int32(0);
elseif jump < -1000
    offset = int32(1023);
end

% We record the last input BEFORE it's offset. This fixes situations where
% we're comparing data before and after the very first transition.
lastInput = input;

% Apply any offset that should be there.
input = input + offset;

% Update port range limit when the Hall limit switch. Only update to the
% maximum value obtained during the limit switch active period.
if starboard_limit && high_side == -1
    high_side = input;
    
    % If the high_side limit is less than the low_side one, we add 1023
    % assuming that it's a valid value (ie. ~= -1).
    if high_side < low_side && high_side ~= -1
        high_side = high_side + 1023;
    end
    
    if low_side ~= -1
        cal = true;
    end
end

% Update starboard ADC value when limit is reached. Only update to the
% maximum value obtained during the limit switch active period.
if port_limit && low_side == -1
    low_side = input;
    
    % If the high_side limit is less than the low_side one, we add 1023
    % assuming that it's a valid value (ie. ~= -1).
    if high_side < low_side && high_side ~= -1
        high_side = high_side + 1023;
    end
    
    if high_side ~= -1
        cal = true;
    end
end

calibrated = cal;

high_limit = int16(high_side);
low_limit = int16(low_side);

% Return 0 when we can't actually determine the rudder position
if ~cal
    rads = single(0);
    return;
end

% Prepare our input. Here we subtract the baseline 'low_side' value off of
% the input so we start with a range from [0..high_side-lowside] and map it
% into the output range of 45 degrees.
in_max = high_side - low_side;
val = input - low_side;

% Do the actual conversion reversing the range and mapping it into [.7854:-0.7854]
rads = (0.5 - single(val)/single(in_max))*2*0.7854;

% Finally cap the value to +- our range to prevent odd errors later.
if rads > 0.7854
    rads = single(0.7854);
elseif rads < -0.7854
    rads = single(-0.7854);
end

== matlab function Sensor Inputs/Toggle ==
  data: u input double; y output double
function y = toggle(u)
%#eml

persistent pre_output;

% Initialize pre_output
if isempty(pre_output)
    pre_output = false;
end

% If we receive the toggle input, toggle
if u
    if pre_output
        pre_output = false;
    else
        pre_output = true;
    end
end

y = pre_output;

== matlab function Controller/Radio Control Inputs1/Detect calibration trigger/Compute Calibration State ==
  data: trigger input boolean; state output uint8; restoredCalibration input double
function state = fcn(trigger, restoredCalibration)
%#eml

persistent countdownTimer transitionCounter internalState;

% Initialize persistent variables
if isempty(countdownTimer)
    countdownTimer = uint8(0);
    transitionCounter = uint8(0);
    
    if restoredCalibration
        internalState = uint8(3);
    else
        internalState = uint8(0);
    end
end

% Do the state processing:
switch internalState
    case 0 % Off
        % When we get a trigger, go into state 1 clearing the timer for use
        if trigger
            transitionCounter = uint8(1);
            internalState = uint8(1);
            countdownTimer = uint8(0);
        end
    case 1 % Transition mode
        % Here we just keep a timer going and once it expires we go back to off,
        % otherwise we count transitions until we've hit 3 then we go to calibration mode.
        countdownTimer = countdownTimer + 1;
        if countdownTimer > 150
            internalState = uint8(0);
        elseif trigger
            transitionCounter = transitionCounter + 1;
        
            % Once we've hit three transitions, we're in calibration mode!
            if transitionCounter == uint8(3)
                internalState = uint8(2);
            end
        end
    case 2 % Calibration mode
        % On the trigger, go into a calibrated mode.
        if trigger
            internalState = uint8(3);
        end
    case 3 % Calibrated
        % When we get a trigger, go into state 4 clearing the timer for use
        if trigger
            transitionCounter = uint8(1);
            internalState = uint8(4);
            countdownTimer = uint8(0);
        end
    case 4 % Transition mode (post-calibration)
        % Here we just keep a timer going and once it expires we go back to calibrated,
        % otherwise we count transitions until we've hit 3 then we go to calibration mode.
        countdownTimer = countdownTimer + 1;
        if countdownTimer > 150
            internalState = uint8(3);
        elseif trigger
            transitionCounter = transitionCounter + 1;
        
            % Once we've hit three transitions, we're in calibration mode!
            if transitionCounter == uint8(3)
                internalState = uint8(2);
            end
        end
end

% Output the internal state
state = internalState;

== matlab function Controller/Select current waypoint track ==
  data: reset output double; nextTrack input double; resetTrackNumber input double; test_waypoints parameter double; figure8_waypoints parameter double; sampling_waypoints parameter double; waypoints output double
function [reset, waypoints] = selectTrack(nextTrack, resetTrackNumber, test_waypoints, figure8_waypoints, sampling_waypoints)
%#eml


% Initialize trackNumber.
% This variable is our state, which is the set of waypoints we're navigating
% between.
persistent trackNumber;
if isempty(trackNumber)
    trackNumber = uint8(1);
end

% Here is the logic for switching tracks. trackReset resets the trackNumber
% and nextTrack increments the track number
if resetTrackNumber
    trackNumber = uint8(1);
    reset = true;
elseif nextTrack
    trackNumber = trackNumber + uint8(1);
    if trackNumber > 3
        trackNumber = uint8(1);
    end
    reset = true;
else
    reset = false;
end

% 1 is for the test waypoints, 2 is for the figure eight, and 3 is
% for the data gathering waypoints.
switch trackNumber
    case 1
        waypoints = test_waypoints;
    case 2
        waypoints = figure8_waypoints;
    case 3
        waypoints = sampling_waypoints;
    otherwise
        waypoints = zeros(size(test_waypoints), 'int32');
end

== matlab function Transmit state data via UART1/Pack1 ==
  data: L2 input double; gPos input double; head input double; lPos input double; vel input double; wp0 input double; wp1 input double; y output double; rudder_pot input double; port_limit input double; sb_limit input double; lat input double; lon input double; alt input double; yr input double; mon input double; day input double; hr input double; min input double; sec input double; cog input double; sog input double; hdop input double; fix input double; sat input double; reset input double; load input double; rudder_angle input double; v_rpm input double; status input double; ordering input double; rudderAngleCommand input double; throttleCommand input double; batteryVoltage input double; batteryAmperage input double; lowRudderCalLimit input double; highRudderCalLimit input double
function y = fcn(L2, gPos, head, lPos, vel, wp0, wp1, rudder_pot, port_limit, sb_limit, lat, lon, alt, yr, mon, day, hr, min, sec, cog, sog, hdop, fix, sat, reset, load, rudder_angle, v_rpm, status, ordering, rudderAngleCommand, throttleCommand, batteryVoltage, batteryAmperage, lowRudderCalLimit, highRudderCalLimit)
%#eml

y = zeros(116, 1, 'uint8');
y(1:4) = packUint32BE(typecast(L2(1),'uint32'));
y(5:8) = packUint32BE(typecast(L2(2),'uint32'));
y(9:12) = packUint32BE(typecast(gPos(1),'uint32'));
y(13:16) = packUint32BE(typecast(gPos(2),'uint32'));
y(17:20) = packUint32BE(typecast(head,'uint32'));
y(21:24) = packUint32BE(typecast(lPos(1),'uint32'));
y(25:28) = packUint32BE(typecast(lPos(2),'uint32'));
y(29:32) = packUint32BE(typecast(vel(1),'uint32'));
y(33:36) = packUint32BE(typecast(vel(2),'uint32'));
y(37:40) = packUint32BE(typecast(wp0(1),'uint32'));
y(41:44) = packUint32BE(typecast(wp0(2),'uint32'));
y(45:48) = packUint32BE(typecast(wp1(1),'uint32'));
y(49:52) = packUint32BE(typecast(wp1(2),'uint32'));
y(53:54) = packUint16BE(rudder_pot);
y(55) = port_limit;
y(56) = sb_limit;
y(57:60) = packUint32BE(typecast(lat,'uint32'));
y(61:64) = packUint32BE(typecast(lon,'uint32'));
y(65:68) = packUint32BE(typecast(alt,'uint32'));
y(69) = yr;
y(70) = mon;
y(71) = day;
y(72) = hr;
y(73) = min;
y(74) = sec;
y(75:78) = packUint32BE(typecast(cog,'uint32'));
y(79:82) = packUint32BE(typecast(sog,'uint32'));
y(83:86) = packUint32BE(typecast(hdop,'uint32'));
y(87) = fix;
y(88) = sat;
y(89) = reset;
y(90) = load;
y(91:94) = packUint32BE(typecast(rudder_angle,'uint32'));
y(95:96) = packUint16BE(typecast(v_rpm,'uint16'));
y(97) = status;
y(98) = ordering;
y(99:102) = packUint32BE(typecast(rudderAngleCommand,'uint32'));
y(103:104) = packUint16BE(typecast(throttleCommand, 'uint16'));
y(105:108) = packUint32BE(typecast(batteryVoltage,'uint32'));
y(109:112) = packUint32BE(typecast(batteryAmperage,'uint32'));
y(113:114) = packUint16BE(typecast(lowRudderCalLimit, 'uint16'));
y(115:116) = packUint16BE(typecast(highRudderCalLimit, 'uint16'));

function out = packUint32BE(in)
out = zeros(4, 1, 'uint8');
out(1) = uint8(bitand(bitshift(in,-24),hex2dec('FF')));
out(2) = uint8(bitand(bitshift(in,-16),hex2dec('FF')));
out(3) = uint8(bitand(bitshift(in,-8),hex2dec('FF')));
out(4) = uint8(bitand(in,hex2dec('FF')));

function out = packUint16BE(in)
out = zeros(2, 1, 'uint8');
out(1) = uint8(bitand(bitshift(in,-8),hex2dec('FF')));
out(2) = uint8(bitand(in,hex2dec('FF')));

== matlab function Controller/Radio Control Inputs1/If Action Subsystem1/Map into range ==
  data: mappedValue output int32; val input int32; in_min input int32; in_max input int32; out_min input int32; out_max input int32
function mappedValue = map(val, in_min, in_max, out_min, out_max)
%#eml
% Pulled from: http://www.arduino.cc/cgi-bin/yabb2/YaBB.pl?num=1289758376, first post
% This is a basic integer implementation of a map() function.
% NOTE: There can be integer overflow in the first multiplication.

  mappedValue = (val - in_min) * (out_max - out_min) / (in_max - in_min) + out_min;

end

== matlab function Controller/Radio Control Inputs1/If Action Subsystem3/Map into range ==
  data: mappedValue output int32; val input int32; in_min input int32; in_max input int32; out_min input int32; out_max input int32
function mappedValue = map(val, in_min, in_max, out_min, out_max)
%#eml
% Pulled from: http://www.arduino.cc/cgi-bin/yabb2/YaBB.pl?num=1289758376, first post
% This is a basic integer implementation of a map() function.
% NOTE: There can be integer overflow in the first multiplication.

  mappedValue = (val - in_min) * (out_max - out_min) / (in_max - in_min) + out_min;

end

== matlab function Controller/Radio Control Inputs1/If Action Subsystem5/Map into range ==
  data: mappedValue output int32; val input int32; in_min input int32; in_max input int32; out_min input int32; out_max input int32
function mappedValue = map(val, in_min, in_max, out_min, out_max)
%#eml
% Pulled from: http://www.arduino.cc/cgi-bin/yabb2/YaBB.pl?num=1289758376, first post
% This is a basic integer implementation of a map() function.
% NOTE: There can be integer overflow in the first multiplication.

  mappedValue = (val - in_min) * (out_max - out_min) / (in_max - in_min) + out_min;

end

== matlab function Controller/Autonomous Controller/Throttle Command/Mux Everything/Select data packet ==
  data: y output double; dis input double; en input double
function y = fcn(dis, en)
% This block controls the switch selecting between enable, 
% disable, and speed commands. If disable and enable are
% both set high, disable overrides anything else.

y = uint8(3);
if dis == 1
    y = uint8(1);
elseif en == 1
    y = uint8(2);
end

== matlab function Transmit state data via UART1/Build HIL sentence/Pack ==
  data: a input double; y output double; b input double; c input double; d input double; e input double; f input double
function y = fcn(a, b, c, d, e, f)
%#eml

y = zeros(length(a)+length(b)+length(c)+length(d)+length(e)+length(f), 1, 'uint8');
y(1) = a;
y(2) = b;
y(3:120) = c;
y(121) = d;
y(122) = e;
y(123) = f;

== matlab function Controller/Radio Control Inputs1/autoMode State Checker ==
  data: rcInput input double; y output double; HIL input double
function y  = fcn(rcInput, HIL)
%#eml

% Initialize a persistent state variable that initializes to -1, the startup
% state value.
persistent internalState;
if isempty(internalState)
    internalState = int8(-1);
end

% Implement the state machine.
switch internalState
    case -1 % Startup
        if rcInput ~= 0
            if rcInput > 7000
                internalState = int8(0);
            else
                internalState = int8(1);
            end
        elseif HIL
            internalState = int8(1);
        end
    case 0 % Manual mode
        if rcInput ~= 0
            if rcInput > 7000
                internalState = int8(0);
            else
                internalState = int8(1);
            end
        elseif HIL
            internalState = int8(1);
        end
    case 1 % Autonomous mode
        if rcInput ~= 0
            if rcInput > 7000
                internalState = int8(0);
            else
                internalState = int8(1);
            end
        end
end
    
% Here the current autonomous state is output as either 1:"on" or 0:"off"
if internalState == int8(1)
    y = true;
else
    y = false;
end
